simulink model "DCmotormodelWindUpFF"  (R2024b)
settings: Solver=VariableStepAuto  StartTime=0.0  StopTime=18  MaxStep=1e-4  RelTol=1e-4  AbsTol=1e-5
values from neighbouring files (symbols this model uses):
  ilim = 1*Ia_nom    (= 3.65)    [DCMOTORELAST.m]    (also in simulazione_vuota1.mat = 4.38; simulazione_vuota2lim.mat = 4.38)
  kamp = Va_lim/dcvolt    (= 5.76)    [DCMOTORELAST.m]    (also in simulazione_vuota1.mat; simulazione_vuota2lim.mat)
  kdt = Vctr/omega_max_rad    (= 0.0131293711322)    [DCMOTORELAST.m]    (also in simulazione_vuota1.mat = 0.0131278037994; simulazione_vuota2lim.mat = 0.0131278037994)
  kff = kv/(kamp*kdt)    (= 0.921781173607)    [DCMOTORELAST.m]
  ki = Ki_opt    (= 56)    [DCMOTORELAST.m]
  klim_corr = dcvolt/(0.2*Ia_nom)    (= 6.84931506849)    [DCMOTORELAST.m]    (also in simulazione_vuota1.mat; simulazione_vuota2lim.mat)
  kp = kpf    [DCMOTORELAST.m]
  kt = kv    (= 0.0697098650743)    [DCMOTORELAST.m]    (also in simulazione_vuota1.mat = 0.0697; simulazione_vuota2lim.mat = 0.0697)
  kv = kvC*60/(1000*2*pi)    (= 0.0697098650743)    [DCMOTORELAST.m]    (also in simulazione_vuota1.mat = 0.0697; simulazione_vuota2lim.mat = 0.0697)
  S_wu = 1.2*(Ra*Iamax/kamp)    (= 0.387156307417)    [DCMOTORELAST.m]
  Va_lim = 1.2*Va_nom    (= 28.8)    [DCMOTORELAST.m]    (also in simulazione_vuota1.mat; simulazione_vuota2lim.mat)
  Vctr = Va/kamp    (= 4.12471358951)    [DCMOTORELAST.m]    (also in simulazione_vuota1.mat = 4.12422119268; simulazione_vuota2lim.mat = 4.12422119268)
libraries: cstblocks x2
settings Model: Creator=marco  LastModifiedBy=david

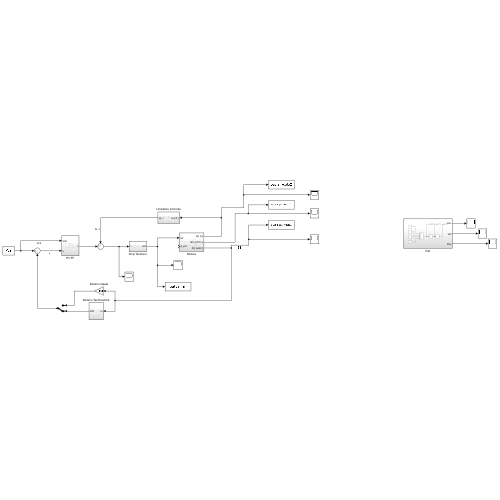
[thumbnail: Simulink's stored preview of the top-level diagram]
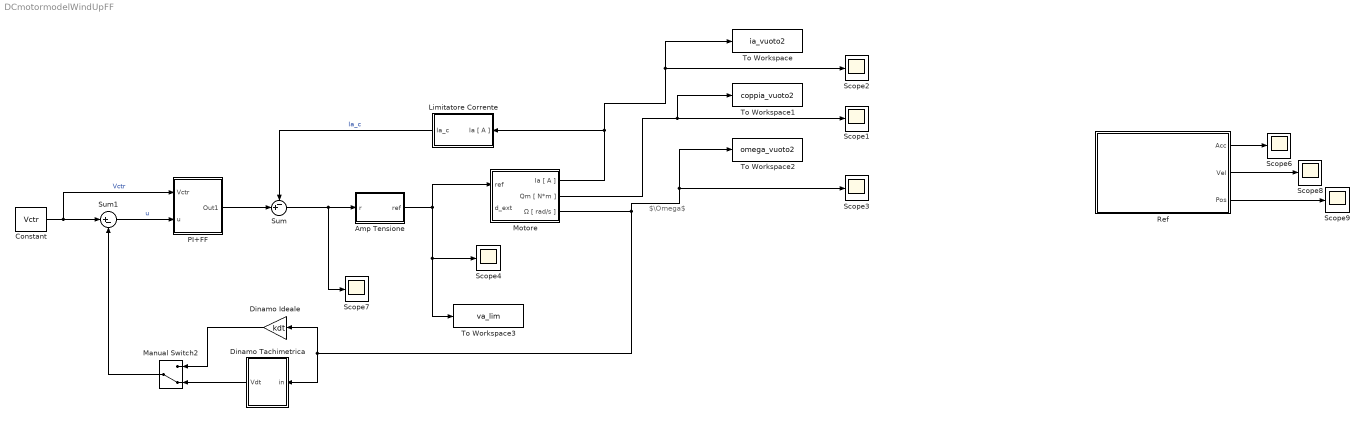
== system DCmotormodelWindUpFF ==
  note: $\Omega$
  Amp Tensione : Subsystem
  Constant : Constant  Value=Vctr
  Dinamo Ideale : Gain  Gain=kdt
  Dinamo Tachimetrica : Subsystem
  Limitatore Corrente : Subsystem
  Manual Switch2 : ManualSwitch  CurrentSetting=0
  Motore : Subsystem
  PI+FF : Subsystem
  Ref : Subsystem
  Scope{1..4,6..9} (8 alike) : Scope
  Sum : Sum  Inputs=-+|
  Sum1 : Sum  Inputs=|+-
  To Workspace : ToWorkspace  VariableName=ia_vuoto2  SaveFormat=Timeseries  SampleTime=-1
  To Workspace1 : ToWorkspace  VariableName=coppia_vuoto2  SaveFormat=Timeseries  SampleTime=-1
  To Workspace2 : ToWorkspace  VariableName=omega_vuoto2  SaveFormat=Timeseries  SampleTime=-1
  To Workspace3 : ToWorkspace  VariableName=va_lim  SaveFormat=Timeseries  SampleTime=-1
  wires:
  Motore/1(Ia [ A ]) -> To Workspace/1, Scope2/1, Limitatore Corrente/1(Ia [ A ])
  Motore/2(Qm [ N*m ]) -> To Workspace1/1, Scope1/1
  Motore/3(Ω [ rad/s ]) -> To Workspace2/1, Scope3/1, Dinamo Tachimetrica/1(in), Dinamo Ideale/1
  Amp Tensione/1(ref) -> Motore/1(ref), Scope4/1, To Workspace3/1
  Sum/1 -> Amp Tensione/1(r), Scope7/1
  Limitatore Corrente/1(Ia_c) -> Sum/1  "Ia_c"
  Dinamo Tachimetrica/1(Vdt) -> Manual Switch2/2
  Manual Switch2/1 -> Sum1/2
  Dinamo Ideale/1 -> Manual Switch2/1
  Constant/1 -> PI+FF/1(Vctr), Sum1/1  "Vctr"
  Sum1/1 -> PI+FF/2(u)  "u"
  PI+FF/1(Out1) -> Sum/2
  Ref/1(Acc) -> Scope6/1
  Ref/2(Vel) -> Scope8/1
  Ref/3(Pos) -> Scope9/1

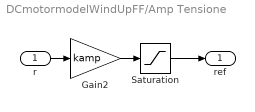
== system DCmotormodelWindUpFF/Amp Tensione ==
  r : Inport
  Gain2 : Gain  Gain=kamp
  Saturation : Saturate  UpperLimit=Va_lim  LowerLimit=-Va_lim
  ref : Outport
  wires:
  Saturation/1 -> ref/1
  Gain2/1 -> Saturation/1
  r/1 -> Gain2/1

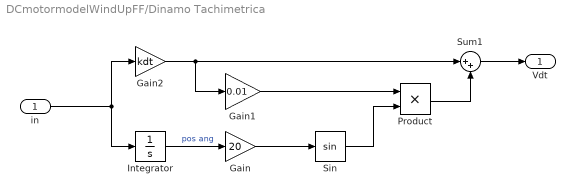
== system DCmotormodelWindUpFF/Dinamo Tachimetrica ==
  in : Inport
  Gain : Gain  Gain=20
  Gain1 : Gain  Gain=0.01
  Gain2 : Gain  Gain=kdt
  Integrator : Integrator
  Product : Product
  Sin : Trigonometry
  Sum1 : Sum  Inputs=|++
  Vdt : Outport
  wires:
  Integrator/1 -> Gain/1  "pos ang"
  Sum1/1 -> Vdt/1
  Gain/1 -> Sin/1
  Gain2/1 -> Gain1/1, Sum1/1
  Gain1/1 -> Product/1
  in/1 -> Integrator/1, Gain2/1
  Product/1 -> Sum1/2
  Sin/1 -> Product/2

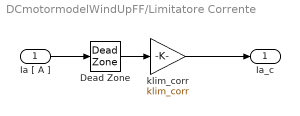
== system DCmotormodelWindUpFF/Limitatore Corrente ==
  Ia [ A ] : Inport
  Dead Zone : DeadZone  LowerValue=-ilim  UpperValue=ilim
  klim_corr : Gain  Gain=klim_corr
  Ia_c : Outport
  wires:
  Ia [ A ]/1 -> Dead Zone/1
  Dead Zone/1 -> klim_corr/1
  klim_corr/1 -> Ia_c/1

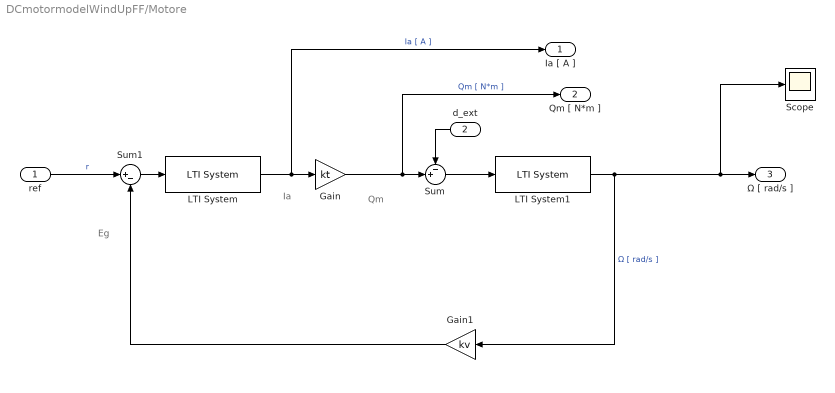
== system DCmotormodelWindUpFF/Motore ==
  note: Qm
  note: Ia
  note: Eg
  ref : Inport
  d_ext : Inport  Port=2
  Gain : Gain  Gain=kt
  Gain1 : Gain  Gain=kv
  LTI System : cstblocks/LTI System  sys=P_el  IC=[]  PadeOrder=0
  LTI System1 : cstblocks/LTI System  sys=P_mec  IC=[]  PadeOrder=0
  Scope : Scope
  Sum : Sum  Inputs=-+|
  Sum1 : Sum  Inputs=|+-
  Ia [ A ] : Outport
  Qm [ N*m ] : Outport  Port=2
  Ω [ rad/s ] : Outport  Port=3
  wires:
  Gain/1 -> Qm [ N*m ]/1, Sum/2  "Qm [ N*m ]"
  Sum/1 -> LTI System1/1
  Gain1/1 -> Sum1/2
  Sum1/1 -> LTI System/1
  LTI System1/1 -> Scope/1, Ω [ rad/s ]/1, Gain1/1  "Ω [ rad/s ]"
  LTI System/1 -> Ia [ A ]/1, Gain/1  "Ia [ A ]"
  ref/1 -> Sum1/1  "r"
  d_ext/1 -> Sum/1

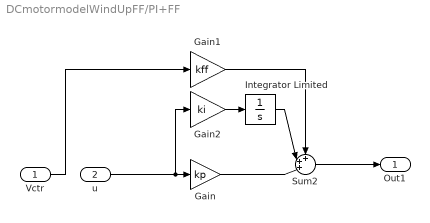
== system DCmotormodelWindUpFF/PI+FF ==
  Vctr : Inport
  u : Inport  Port=2
  Gain : Gain  Gain=kp
  Gain1 : Gain  Gain=kff
  Gain2 : Gain  Gain=ki
  Integrator Limited : Integrator  LimitOutput=on  UpperSaturationLimit=S_wu  LowerSaturationLimit=-S_wu
  Sum2 : Sum  Inputs=+++|
  Out1 : Outport
  wires:
  Integrator Limited/1 -> Sum2/2
  Gain/1 -> Sum2/3
  u/1 -> Gain2/1, Gain/1
  Vctr/1 -> Gain1/1
  Gain2/1 -> Integrator Limited/1
  Gain1/1 -> Sum2/1
  Sum2/1 -> Out1/1

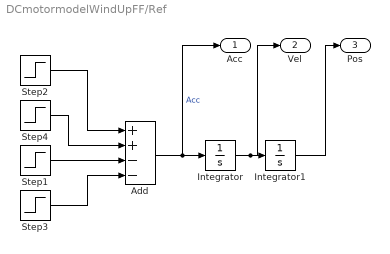
== system DCmotormodelWindUpFF/Ref ==
  Add : Sum  Inputs=++--
  Integrator : Integrator
  Integrator1 : Integrator
  Step1 : Step  Time=2.5  After=209.33  SampleTime=0
  Step2 : Step  After=209.33  SampleTime=0
  Step3 : Step  Time=14.5  After=209.33  SampleTime=0
  Step4 : Step  Time=16  After=209.33  SampleTime=0
  Acc : Outport
  Vel : Outport  Port=2
  Pos : Outport  Port=3
  wires:
  Step2/1 -> Add/1
  Step3/1 -> Add/4
  Integrator1/1 -> Pos/1
  Step1/1 -> Add/3
  Step4/1 -> Add/2
  Integrator/1 -> Vel/1, Integrator1/1
  Add/1 -> Acc/1, Integrator/1  "Acc"
